simulink model "Tecsys2"  (R2022b)
settings: Solver=ode45  StartTime=0.0  StopTime=inf  RelTol=1e-3  EnableMultiTasking=on
undefined symbols (not defined in the file): qpsktxrx
libraries: commrandsrc3 x2, commdigbbndpm3 x2, commfilt2 x2, commchan3 x1, commsink2 x1, commsync2 x1, simulink x1, dspsigops x1
settings Model: Creator=The MathWorks, Inc.  LastModifiedBy=Leoni Gabriel
settings SolverCC: AlgebraicLoopSolver=TrustRegion
settings DataIOCC: LimitDataPoints=on  SaveFormat=Array  ReturnWorkspaceOutputs=off
settings OptimizationCC: LifeSpan=inf
settings DebuggingCC: SolverPrmCheckMsg=warning  UnconnectedInputMsg=warning  UnconnectedOutputMsg=warning  UnconnectedLineMsg=warning  AllowSymbolicDim=off  SFUnexpectedBacktrackingDiag=warning  SFNoUnconditionalDefaultTransitionDiag=warning  SFExecutionAtInitializationDiag=none  SFMachineParentedDataDiag=warning  ArithmeticOperatorsInVariantConditions=warning
settings HardwareCC: ProdBitPerPointer=32  ProdBitPerSizeT=32  ProdBitPerPtrDiffT=32  ProdLargestAtomicFloat=None  ProdIntDivRoundTo=Undefined  ProdEndianess=Unspecified  ProdWordSize=32  ProdHWDeviceType=32-bit Generic
settings ModelReferenceCC: EnableRefExpFcnMdlSchedulingChecks=on  PropagateSignalLabelsOutOfModel=off
settings SFSimCC: SimUseLocalCustomCode=off
settings RTWCC: RTWUseLocalCustomCode=off  DLArmComputeVersion=19.05
settings CodeAppCC: StateflowObjectComments=on
settings GRTTargetCC: TargetLangStandard=C89/C90 (ANSI)
settings ConfigComp: CovMetricSettings=dw  CovSaveCumulativeToWorkspaceVar=on  CovSaveSingleToWorkspaceVar=on  CovExternalEMLEnable=off  CovSFcnEnable=off

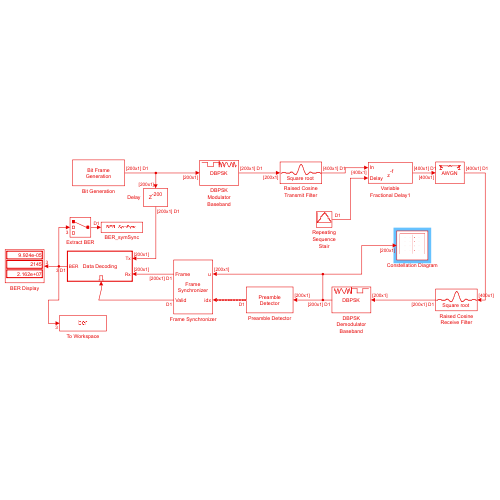
[thumbnail: Simulink's stored preview of the top-level diagram]
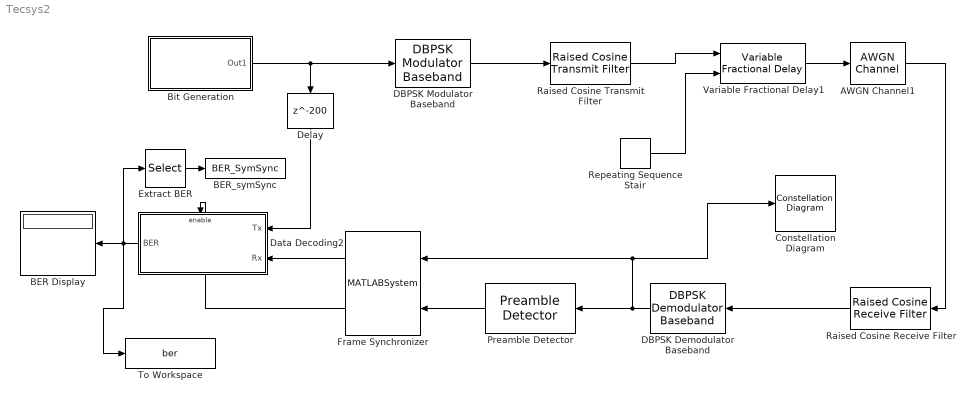
== system Tecsys2 ==
  AWGN Channel1 : commchan3/AWGN Channel  InputProcessing=Columns as channels (frame based)  seed=67  noiseMode="Signal to noise ratio  (SNR)"  EbNodB=7  EsNodB=15  SNRdB=40  bitsPerSym=2  Ps=1/2  Tsym=qpsktxrx.Upsampling*qpsktxrx.Ts  variance=1
  BER Display : Display
  BER_symSync : ToWorkspace  VariableName=BER_SymSync  SaveFormat=Timeseries  SampleTime=-1
  Bit Generation : Subsystem
      mask Display: disp('Bit Frame\nGeneration')
  Constellation Diagram : ConstellationDiagram  WindowPosition=[186.000000,12.000000,683.000000,705.000000,]  ScopeFrameLocation=window  SamplesPerSymbol=2  XLimits=[-1.39,1.39]  YLimits=[-1.38,1.38]  ShowLegend=on
  DBPSK Demodulator Baseband : commdigbbndpm3/DBPSK Demodulator Baseband  Ph=0  outDtype=Inherit via internal rule
  DBPSK Modulator Baseband : commdigbbndpm3/DBPSK Modulator Baseband  Ph=0  outDtype=double
  Data Decoding2 : Subsystem
      mask Display: disp('Data Decoding');
  Delay : Delay  DelayLength=200  InputProcessing=Columns as channels (frame based)  UseCircularBuffer=on
  Extract BER : Selector  InputPortWidth=3  IndexOptions=Index vector (dialog)  Indices=1  OutputSizes=1
  Frame Synchronizer : MATLABSystem  System=comm.internal.examples.FrameSynchronizer  Input=Bit  OutputFrameLength=200  PreambleLength=40  SimulateUsing=Code generation
      mask Type: comm.internal.examples.FrameSynchronizer
      mask Display:
      | disp(['Frame' char(10) 'Synchronizer']);
      | port_label('input',1,'u');
      | port_label('input',2,'idx');
      | port_label('output',1,'Frame');
      | port_label('output',2,'Valid');
  Preamble Detector : commsync2/Preamble Detector  Input=Bit  Preamble=[1 0 0 1 0 1 1 0 1 1 1 0 1 0 1 1 0 1 1 0 1 0 0 1 0 1 1 0 1 1 1 0 1 0 1 1 0 1 1 0]'  Threshold=3  DetectionMetricOutput=off  Detections=First  SimulateUsing=Code generation
  Raised Cosine Receive Filter : commfilt2/Raised Cosine Receive Filter  filtType=Square root  R=0.5  filtSpan=10  N=2  downFactor=2  downOffset=0  filterGain=1  InputProcessing=Columns as channels (frame based)  RateOptions=Enforce single-rate processing  framing=Mute  checkCoeff=off  variableName=rcRxFilt  currentFiltSpan=10  D=5  inputOffset=0  sampMode=Mute  saveAsFlag=0  rateMode=Downsampling  checkGain=Normalized  launchFVT=on  roundingMode=Floor  overflowMode=off  coeffDataTypeStr=Inherit: Same word length as input  coeffMin=[]  coeffMax=[]  coeffLastDataTypeStr=Inherit: Same word length as input  accumDataTypeStr=Inherit: Same as product output  accumLastDataTypeStr=Inherit: Same as product output  outputDataTypeStr=Inherit: Same as accumulator  outputMin=[]  outputMax=[]  outputLastDataTypeStr=Inherit: Same as accumulator
  Raised Cosine Transmit Filter : commfilt2/Raised Cosine Transmit Filter  filtType=Square root  R=0.5  filtSpan=10  N=2  filterGain=1  InputProcessing=Columns as channels (frame based)  RateOptions=Enforce single-rate processing  framing=Mute  checkCoeff=off  variableName=rcTxFilt  checkGain=Normalized  sampMode=Mute  saveAsFlag=0  currentFiltSpan=10  D=(10)/2  launchFVT=on  roundingMode=Floor  overflowMode=off  coeffDataTypeStr=Inherit: Same word length as input  coeffMin=[]  coeffMax=[]  coeffLastDataTypeStr=Inherit: Same word length as input  outputDataTypeStr=Inherit: Same as accumulator  outputMin=[]  outputMax=[]  outputLastDataTypeStr=Inherit: Same as accumulator
  Repeating Sequence Stair : simulink/Sources/Repeating Sequence Stair  OutValues=[0:0.1:0.9 0.8:-0.1:0.1]  tsamp=-1  OutMin=[]  OutMax=[]  OutDataTypeStr=double  OutputDataTypeScalingMode=double  OutDataType=fixdt(0,8)  ConRadixGroup=Best Precision: Vector-wise  OutScaling=2^-12
  To Workspace : ToWorkspace  VariableName=ber  SaveFormat=Timeseries  SampleTime=-1
  Variable Fractional Delay1 : dspsigops/Variable Fractional Delay  mode=OBSOLETE  modeActive=Linear  L=4  FarrowL=4  R=10  alpha=1  dmax=400  InputProcessing=Columns as channels (frame based)  ic=0  noDFT=off  fallbackFIR=Clip to the minimum value necessary for centered kernel  fallbackFarrow=Clip to the minimum value necessary for centered kernel  roundingMode=Zero  overflowMode=off
  wires:
  Bit Generation/1(Out1) -> DBPSK Modulator Baseband/1, Delay/1
  Preamble Detector/1 -> Frame Synchronizer/2
  DBPSK Demodulator Baseband/1 -> Constellation Diagram/1, Frame Synchronizer/1, Preamble Detector/1
  Frame Synchronizer/1 -> Data Decoding2/2(Rx)
  Frame Synchronizer/2 -> Data Decoding2/Enable
  Delay/1 -> Data Decoding2/1(Tx)
  Extract BER/1 -> BER_symSync/1
  Data Decoding2/1(BER) -> Extract BER/1, BER Display/1, To Workspace/1
  DBPSK Modulator Baseband/1 -> Raised Cosine Transmit Filter/1
  AWGN Channel1/1 -> Raised Cosine Receive Filter/1
  Repeating Sequence Stair/1 -> Variable Fractional Delay1/2
  Raised Cosine Transmit Filter/1 -> Variable Fractional Delay1/1
  Variable Fractional Delay1/1 -> AWGN Channel1/1
  Raised Cosine Receive Filter/1 -> DBPSK Demodulator Baseband/1

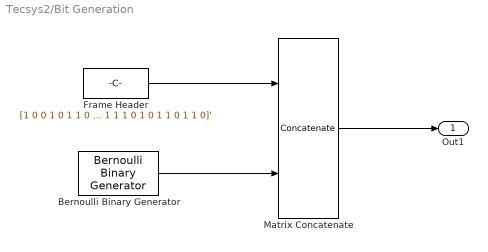
== system Tecsys2/Bit Generation ==
  Bernoulli Binary Generator : commrandsrc3/Bernoulli Binary Generator  ProbabilityOfZero=0.5  SeedSource=Parameter  Seed=61  SampleTime=1  SamplesPerFrame=160  OutputDataType=double  SimulateUsing=Interpreted execution
  Frame Header : Constant  Value=[1 0 0 1 0 1 1 0 1 1 1 0 1 0 1 1 0 1 1 0 1 0 0 1 0 1 1 0 1 1 1 0 1 0 1 1 0 1 1 0]'  VectorParams1D=off  OutDataTypeStr=double
  Matrix Concatenate : Concatenate  Mode=Multidimensional array
  Out1 : Outport  VectorParamsAs1DForOutWhenUnconnected=off
  wires:
  Matrix Concatenate/1 -> Out1/1
  Frame Header/1 -> Matrix Concatenate/1
  Bernoulli Binary Generator/1 -> Matrix Concatenate/2

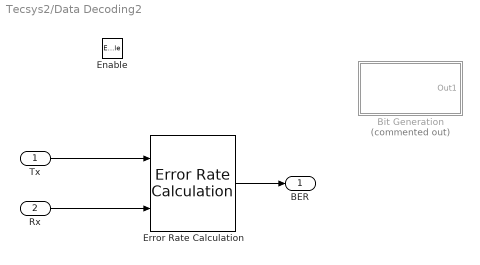
== system Tecsys2/Data Decoding2 ==
  Tx : Inport
  Rx : Inport  Port=2
  Enable : EnablePort
  Bit Generation : Subsystem  Commented=on
      mask Display: disp('Bit Frame\nGeneration')
  Error Rate Calculation : commsink2/Error Rate Calculation  N=0  st_delay=0  cp_mode=Entire frame  subframe=[]  PMode=Port  WsName=ErrorVec  RsMode2=off  stop=off  numErr=100  maxBits=1e6
  BER : Outport  VectorParamsAs1DForOutWhenUnconnected=off
  wires:
  Error Rate Calculation/1 -> BER/1
  Rx/1 -> Error Rate Calculation/2
  Tx/1 -> Error Rate Calculation/1

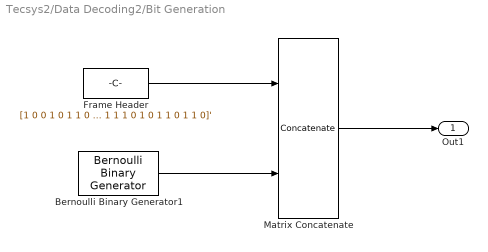
== system Tecsys2/Data Decoding2/Bit Generation ==
  Bernoulli Binary Generator1 : commrandsrc3/Bernoulli Binary Generator  ProbabilityOfZero=0.5  SeedSource=Parameter  Seed=61  SampleTime=1  SamplesPerFrame=160  OutputDataType=double  SimulateUsing=Interpreted execution
  Frame Header : Constant  Value=[1 0 0 1 0 1 1 0 1 1 1 0 1 0 1 1 0 1 1 0 1 0 0 1 0 1 1 0 1 1 1 0 1 0 1 1 0 1 1 0]'  VectorParams1D=off  OutDataTypeStr=double
  Matrix Concatenate : Concatenate  Mode=Multidimensional array
  Out1 : Outport  VectorParamsAs1DForOutWhenUnconnected=off
  wires:
  Matrix Concatenate/1 -> Out1/1
  Frame Header/1 -> Matrix Concatenate/1
  Bernoulli Binary Generator1/1 -> Matrix Concatenate/2
